simulink model "MdEnChk6s7s_LugALL"  (R2018b)
settings: Solver=FixedStepDiscrete  StartTime=0.0  StopTime=10.0  FixedStep=0.01  RelTol=1e-3
settings Model: Creator=sn2xws  LastModifiedBy=sn2xws
settings DataIOCC: SaveFormat=StructureWithTime
settings OptimizationCC: DefaultParameterBehavior=Inlined  EnhancedBackFolding=on  PassReuseOutputArgsAs=Individual arguments  ZeroExternalMemoryAtStartup=off  ZeroInternalMemoryAtStartup=off  OptimizeBlockOrder=speed  DifferentSizesBufferReuse=on  OptimizationCustomize=off
settings DebuggingCC: ParameterTunabilityLossMsg=error
settings ModelReferenceCC: ModelReferenceNumInstancesAllowed=Single
settings SFSimCC: MATLABDynamicMemAlloc=off
settings RTWCC: SystemTargetFile=autosar.tlc  GenCodeOnly=on  TemplateMakefile=ert_default_tmf  Description=AUTOSAR  GenerateReport=on  IncludeHyperlinkInReport=on  LaunchReport=on  GenerateTraceInfo=on  GenerateTraceReport=on  GenerateTraceReportSl=on  GenerateTraceReportSf=on  GenerateTraceReportEml=on
settings CodeAppCC: ForceParamTrailComments=on  IgnoreCustomStorageClasses=off  OperatorAnnotations=on  SimulinkDataObjDesc=on  SFDataObjDesc=on  InsertBlockDesc=on
settings STFCustomTargetCC: TargetLangStandard=C99 (ISO)  MultiwordLength=256  ParMdlRefBuildCompliant=on  CompOptLevelCompliant=on  IncludeMdlTerminateFcn=off  CombineOutputUpdateFcns=on  SuppressErrorStatus=on  ERTCustomFileBanners=on  SupportNonFinite=off  SupportComplex=off  SupportContinuousTime=off  SupportNonInlinedSFcns=off  RemoveResetFunc=on  MATLABClassNameForMDSCustomization=Simulink.SoftwareTarget.ERTCustomization  AutosarCompliant=on  UseToolchainInfoCompliant=on  LookupTableObjectStructAxisOrder=2,1,3,4,...  LUTObjectStructOrderEvenSpacing=Size,Table,Breakpoints  SystemTargetFile=autosar.tlc
settings ERTTargetCC: TargetLangStandard=C99 (ISO)  ConcurrentExecutionCompliant=off  IncludeMdlTerminateFcn=off  SuppressErrorStatus=on  SupportNonFinite=off  SupportComplex=off  ModelStepFunctionPrototypeControlCompliant=off  CPPClassGenCompliant=off  AutosarCompliant=on  LookupTableObjectStructAxisOrder=2,1,3,4,...  LUTObjectStructOrderEvenSpacing=Size,Table,Breakpoints  InlinedParameterPlacement=NonHierarchical  ERTCustomFileTemplate=example_file_process.tlc

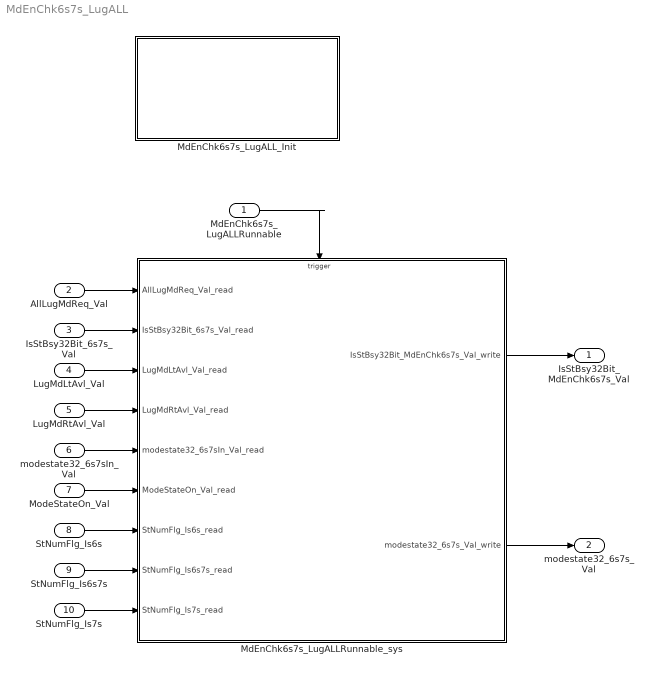
== system MdEnChk6s7s_LugALL ==
  MdEnChk6s7s_LugALLRunnable : Inport  SampleTime=0.01  OutputFunctionCall=on
  AllLugMdReq_Val : Inport  Port=2  OutDataTypeStr=boolean  PortDimensions=1
  IsStBsy32Bit_6s7s_Val : Inport  Port=3  OutDataTypeStr=uint32  PortDimensions=1
  LugMdLtAvl_Val : Inport  Port=4  OutDataTypeStr=boolean  PortDimensions=1
  LugMdRtAvl_Val : Inport  Port=5  OutDataTypeStr=boolean  PortDimensions=1
  modestate32_6s7sIn_Val : Inport  Port=6  OutDataTypeStr=uint32  PortDimensions=1
  ModeStateOn_Val : Inport  Port=7  OutDataTypeStr=boolean  PortDimensions=1
  StNumFlg_Is6s : Inport  Port=8  OutDataTypeStr=boolean  PortDimensions=1
  StNumFlg_Is6s7s : Inport  Port=9  OutDataTypeStr=boolean  PortDimensions=1
  StNumFlg_Is7s : Inport  Port=10  OutDataTypeStr=boolean  PortDimensions=1
  MdEnChk6s7s_LugALLRunnable_sys : Subsystem
  MdEnChk6s7s_LugALL_Init : Subsystem
  IsStBsy32Bit_MdEnChk6s7s_Val : Outport  OutDataTypeStr=uint32  PortDimensions=1
  modestate32_6s7s_Val : Outport  Port=2  OutDataTypeStr=uint32  PortDimensions=1
  wires:
  AllLugMdReq_Val/1 -> MdEnChk6s7s_LugALLRunnable_sys/1(AllLugMdReq_Val_read)
  IsStBsy32Bit_6s7s_Val/1 -> MdEnChk6s7s_LugALLRunnable_sys/2(IsStBsy32Bit_6s7s_Val_read)
  LugMdLtAvl_Val/1 -> MdEnChk6s7s_LugALLRunnable_sys/3(LugMdLtAvl_Val_read)
  LugMdRtAvl_Val/1 -> MdEnChk6s7s_LugALLRunnable_sys/4(LugMdRtAvl_Val_read)
  modestate32_6s7sIn_Val/1 -> MdEnChk6s7s_LugALLRunnable_sys/5(modestate32_6s7sIn_Val_read)
  ModeStateOn_Val/1 -> MdEnChk6s7s_LugALLRunnable_sys/6(ModeStateOn_Val_read)
  StNumFlg_Is6s/1 -> MdEnChk6s7s_LugALLRunnable_sys/7(StNumFlg_Is6s_read)
  StNumFlg_Is6s7s/1 -> MdEnChk6s7s_LugALLRunnable_sys/8(StNumFlg_Is6s7s_read)
  StNumFlg_Is7s/1 -> MdEnChk6s7s_LugALLRunnable_sys/9(StNumFlg_Is7s_read)
  MdEnChk6s7s_LugALLRunnable_sys/1(IsStBsy32Bit_MdEnChk6s7s_Val_write) -> IsStBsy32Bit_MdEnChk6s7s_Val/1
  MdEnChk6s7s_LugALLRunnable_sys/2(modestate32_6s7s_Val_write) -> modestate32_6s7s_Val/1
  MdEnChk6s7s_LugALLRunnable/1 -> MdEnChk6s7s_LugALLRunnable_sys/Trigger

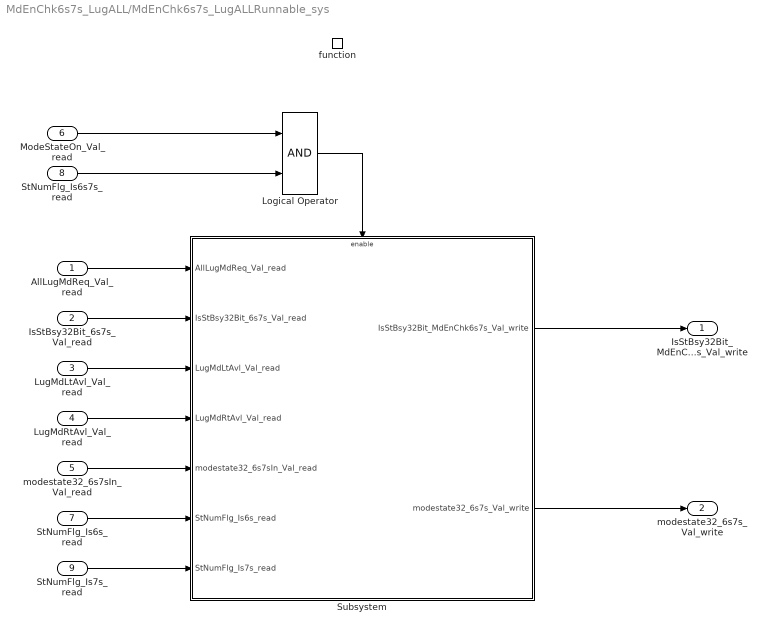
== system MdEnChk6s7s_LugALL/MdEnChk6s7s_LugALLRunnable_sys ==
  AllLugMdReq_Val_read : Inport
  IsStBsy32Bit_6s7s_Val_read : Inport  Port=2
  LugMdLtAvl_Val_read : Inport  Port=3
  LugMdRtAvl_Val_read : Inport  Port=4
  modestate32_6s7sIn_Val_read : Inport  Port=5
  ModeStateOn_Val_read : Inport  Port=6
  StNumFlg_Is6s_read : Inport  Port=7
  StNumFlg_Is6s7s_read : Inport  Port=8
  StNumFlg_Is7s_read : Inport  Port=9
  function : TriggerPort  TriggerType=function-call  VariantControl=(inherit)  SampleTimeType=periodic  SampleTime=-1
  Logical Operator : Logic  AllPortsSameDT=off  OutDataTypeStr=boolean
  Subsystem : Subsystem
  IsStBsy32Bit_MdEnChk6s7s_Val_write : Outport
      settings: EnsureOutportIsVirtual=on
  modestate32_6s7s_Val_write : Outport  Port=2
      settings: EnsureOutportIsVirtual=on
  wires:
  AllLugMdReq_Val_read/1 -> Subsystem/1(AllLugMdReq_Val_read)
  IsStBsy32Bit_6s7s_Val_read/1 -> Subsystem/2(IsStBsy32Bit_6s7s_Val_read)
  LugMdLtAvl_Val_read/1 -> Subsystem/3(LugMdLtAvl_Val_read)
  LugMdRtAvl_Val_read/1 -> Subsystem/4(LugMdRtAvl_Val_read)
  modestate32_6s7sIn_Val_read/1 -> Subsystem/5(modestate32_6s7sIn_Val_read)
  StNumFlg_Is6s_read/1 -> Subsystem/6(StNumFlg_Is6s_read)
  StNumFlg_Is7s_read/1 -> Subsystem/7(StNumFlg_Is7s_read)
  Subsystem/1(IsStBsy32Bit_MdEnChk6s7s_Val_write) -> IsStBsy32Bit_MdEnChk6s7s_Val_write/1
  Subsystem/2(modestate32_6s7s_Val_write) -> modestate32_6s7s_Val_write/1
  StNumFlg_Is6s7s_read/1 -> Logical Operator/2
  Logical Operator/1 -> Subsystem/Enable
  ModeStateOn_Val_read/1 -> Logical Operator/1

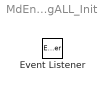
== system MdEnChk6s7s_LugALL/MdEnChk6s7s_LugALL_Init ==
  Event Listener : EventListener  EventName=reset

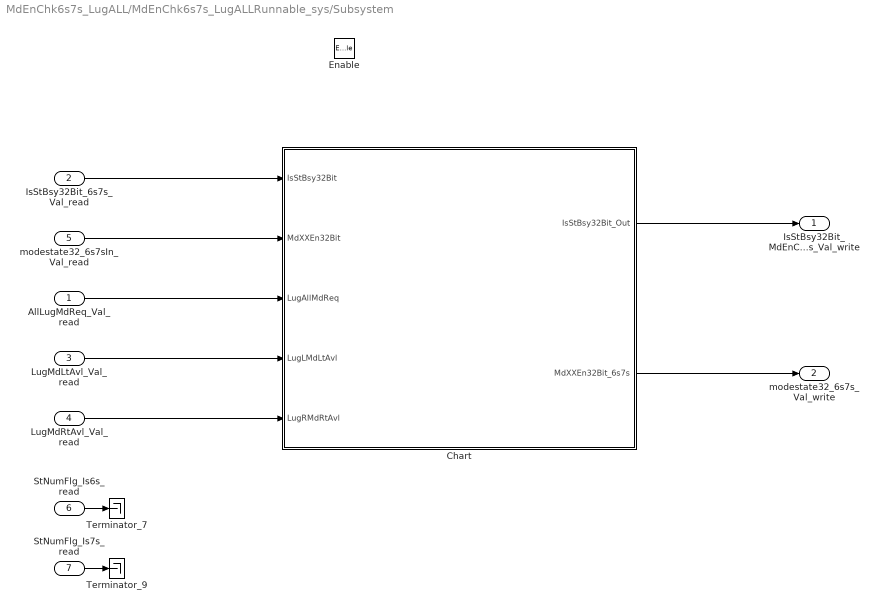
== system MdEnChk6s7s_LugALL/MdEnChk6s7s_LugALLRunnable_sys/Subsystem ==
  AllLugMdReq_Val_read : Inport
  IsStBsy32Bit_6s7s_Val_read : Inport  Port=2
  LugMdLtAvl_Val_read : Inport  Port=3
  LugMdRtAvl_Val_read : Inport  Port=4
  modestate32_6s7sIn_Val_read : Inport  Port=5
  StNumFlg_Is6s_read : Inport  Port=6
  StNumFlg_Is7s_read : Inport  Port=7
  Enable : EnablePort
  Chart : Stateflow chart  TreatAsAtomicUnit=on
  Terminator_7 : Terminator
  Terminator_9 : Terminator
  IsStBsy32Bit_MdEnChk6s7s_Val_write : Outport
      settings: EnsureOutportIsVirtual=on
  modestate32_6s7s_Val_write : Outport  Port=2
      settings: EnsureOutportIsVirtual=on
  wires:
  LugMdLtAvl_Val_read/1 -> Chart/4(LugLMdLtAvl)
  Chart/1(IsStBsy32Bit_Out) -> IsStBsy32Bit_MdEnChk6s7s_Val_write/1
  StNumFlg_Is6s_read/1 -> Terminator_7/1
  StNumFlg_Is7s_read/1 -> Terminator_9/1
  Chart/2(MdXXEn32Bit_6s7s) -> modestate32_6s7s_Val_write/1
  IsStBsy32Bit_6s7s_Val_read/1 -> Chart/1(IsStBsy32Bit)
  modestate32_6s7sIn_Val_read/1 -> Chart/2(MdXXEn32Bit)
  AllLugMdReq_Val_read/1 -> Chart/3(LugAllMdReq)
  LugMdRtAvl_Val_read/1 -> Chart/5(LugRMdRtAvl)

== stateflow chart MdEnChk6s7s_LugALL/MdEnChk6s7s_LugALLRunnable_sys/Subsystem/Chart ==
  state AllMdBsySet [function]
    (default) -> (junction 198)
    (junction 198) -> (junction 199) : {
        | IsStBsy32Bit_Out = IsStBsy32Bit_Out|(EZEBit+EZQBit+VIPLBit+VIPRBit+VIPAllBit+RcvyLBit+RcvyRBit+LugLBit+LugRBit+LugAllBit+FamlyLBit+FamlyRBit+INTMLBit+INTMRBit);
        | }
  (default) -> (junction 44) : {
      | IsStBsy32Bit_Out =IsStBsy32Bit;
      | MdXXEn32Bit_6s7s = MdXXEn32Bit;
      | }
  (junction 44) -> (junction 45) [order 1] : [hasChangedTo(LugAllMdReq,true)&&((MdXXEn32Bit_6s7s&LugAllBit)==0)&&(LugLMdLtAvl||LugRMdRtAvl)]
  (junction 44) -> (junction 46) [order 2]
  (junction 45) -> (junction 47) : {
      | MdXXEn32Bit_6s7s=MdXXEn32Bit_6s7s|(LugLMdLtAvl<<7);
      | MdXXEn32Bit_6s7s =MdXXEn32Bit_6s7s|(LugRMdRtAvl<<8);
      | MdXXEn32Bit_6s7s=MdXXEn32Bit_6s7s|LugAllBit;
      | AllMdBsySet();
      | }
  (junction 47) -> (junction 46)
  (junction 46) -> (junction 48)
  data: IsStBsy32Bit_Out output uint32; MdXXEn32Bit_6s7s output uint32; IsStBsy32Bit input uint32; MdXXEn32Bit input uint32; EZEBit constant uint32 =1; EZQBit constant uint32 =8; VIPAllBit constant uint32 =2; LugAllBit constant uint32 =4; VIPLBit constant uint32 =512; VIPRBit constant uint32 =2048; RcvyLBit constant uint32 =1024; RcvyRBit constant uint32 =4096; INTMLBit constant uint32 =16; INTMRBit constant uint32 =524288; FamlyLBit constant uint32 =64; FamlyRBit constant uint32 =32; LugLBit constant uint32 =128; LugRBit constant uint32 =256; LugAllMdReq input; LugLMdLtAvl input; LugRMdRtAvl input
